simulink model "assgt4_friction"  (R2016a)
settings: Solver=VariableStepAuto  StartTime=0.0  StopTime=30  RelTol=1e-3
values from neighbouring files (symbols this model uses):
  g = 9.81    [assignment4.m]
  l1 = 1    [assignment4.m]
  l2 = 1    [assignment4.m]
  m1 = 1    [assignment4.m]
  m2 = 1    [assignment4.m]
  x_init = [-pi/2;0;0;0]    [assignment4.m]
undefined symbols (not defined in the file or in its folder): x
libraries: dspinverses x1
settings Model: Creator=Sondre  LastModifiedBy=Sondre

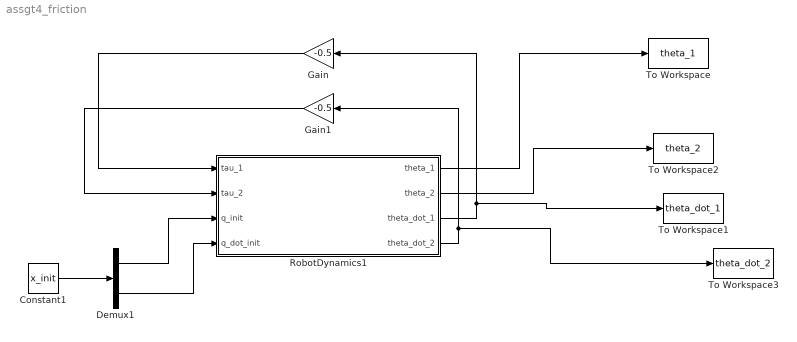
== system assgt4_friction ==
  Constant1 : Constant  Value=x_init
  Demux1 : Demux  Outputs=2
  Gain : Gain  Gain=-0.5
  Gain1 : Gain  Gain=-0.5
  RobotDynamics1 : Subsystem
  To Workspace : ToWorkspace  VariableName=theta_1  SaveFormat=Timeseries  SampleTime=-1
  To Workspace1 : ToWorkspace  VariableName=theta_dot_1  SaveFormat=Timeseries  SampleTime=-1
  To Workspace2 : ToWorkspace  VariableName=theta_2  SaveFormat=Timeseries  SampleTime=-1
  To Workspace3 : ToWorkspace  VariableName=theta_dot_2  SaveFormat=Timeseries  SampleTime=-1
  wires:
  RobotDynamics1/1(theta_1) -> To Workspace/1
  RobotDynamics1/2(theta_2) -> To Workspace2/1
  RobotDynamics1/3(theta_dot_1) -> Gain/1, To Workspace1/1
  RobotDynamics1/4(theta_dot_2) -> Gain1/1, To Workspace3/1
  Constant1/1 -> Demux1/1
  Demux1/1 -> RobotDynamics1/3(q_init)
  Demux1/2 -> RobotDynamics1/4(q_dot_init)
  Gain/1 -> RobotDynamics1/1(tau_1)
  Gain1/1 -> RobotDynamics1/2(tau_2)

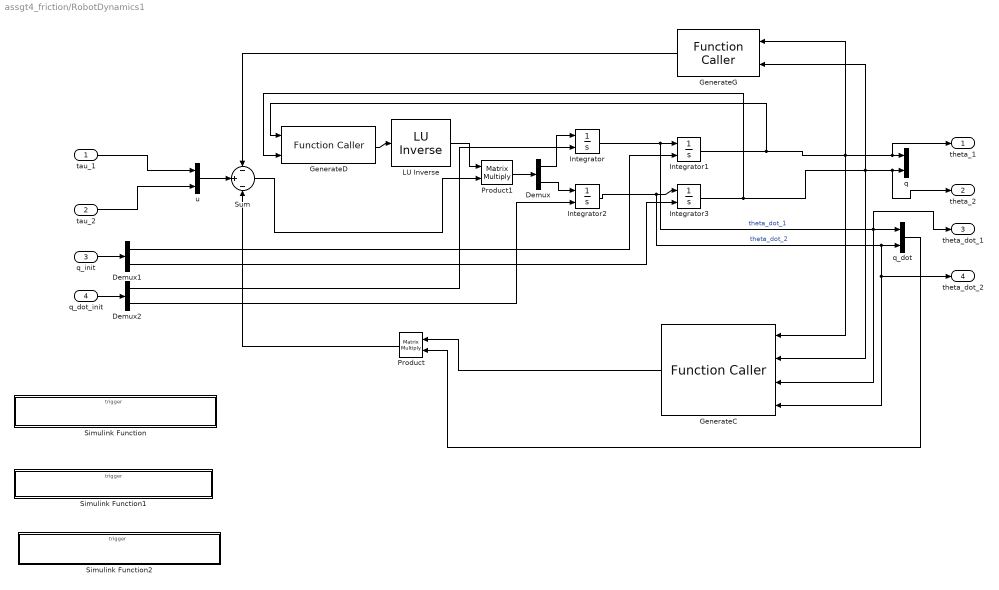
== system assgt4_friction/RobotDynamics1 ==
  tau_1 : Inport
  tau_2 : Inport  Port=2
  q_init : Inport  Port=3
  q_dot_init : Inport  Port=4
  " LU Inverse" : dspinverses/ LU Inverse
  Demux : Demux  Outputs=2
  Demux1 : Demux  Outputs=2
  Demux2 : Demux  Outputs=2
  GenerateC : FunctionCaller  FunctionPrototype=C = C(theta_1,theta_2,theta_dot_1,theta_dot_2)
  GenerateD : FunctionCaller  FunctionPrototype=D = D(theta_1,theta_2)
  GenerateG : FunctionCaller  FunctionPrototype=G = G(theta_1,theta_2)
  Integrator : Integrator  InitialConditionSource=external
  Integrator1 : Integrator  InitialConditionSource=external
  Integrator2 : Integrator  InitialConditionSource=external  InitialCondition=x(
  Integrator3 : Integrator  InitialConditionSource=external
  Product : Product  Multiplication=Matrix(*)
  Product1 : Product  Multiplication=Matrix(*)
  Simulink Function : Subsystem  TreatAsAtomicUnit=on
  Simulink Function1 : Subsystem  TreatAsAtomicUnit=on
  Simulink Function2 : Subsystem  TreatAsAtomicUnit=on
  Sum : Sum  Inputs=-|+|-
  q : Concatenate
  q_dot : Concatenate
  u : Concatenate
  theta_1 : Outport
  theta_2 : Outport  Port=2
  theta_dot_1 : Outport  Port=3
  theta_dot_2 : Outport  Port=4
  wires:
  tau_2/1 -> u/2
  tau_1/1 -> u/1
  u/1 -> Sum/2
  Product/1 -> Sum/3
  q_dot/1 -> Product/2
  GenerateG/1 -> Sum/1
  Sum/1 -> Product1/2
  GenerateC/1 -> Product/1
  GenerateD/1 -> " LU Inverse"/1
  " LU Inverse"/1 -> Product1/1
  Demux/1 -> Integrator/1
  Integrator/1 -> Integrator1/1, q_dot/1, GenerateC/3, theta_dot_1/1  "theta_dot_1"
  Demux/2 -> Integrator2/1
  Integrator2/1 -> GenerateC/4, theta_dot_2/1, q_dot/2, Integrator3/1  "theta_dot_2"
  Product1/1 -> Demux/1
  q_init/1 -> Demux1/1
  q_dot_init/1 -> Demux2/1
  Demux2/1 -> Integrator/2
  Demux2/2 -> Integrator2/2
  Demux1/1 -> Integrator1/2
  Demux1/2 -> Integrator3/2
  Integrator1/1 -> GenerateD/1, theta_1/1, q/1, GenerateG/1, GenerateC/1
  Integrator3/1 -> GenerateD/2, GenerateC/2, GenerateG/2, theta_2/1, q/2

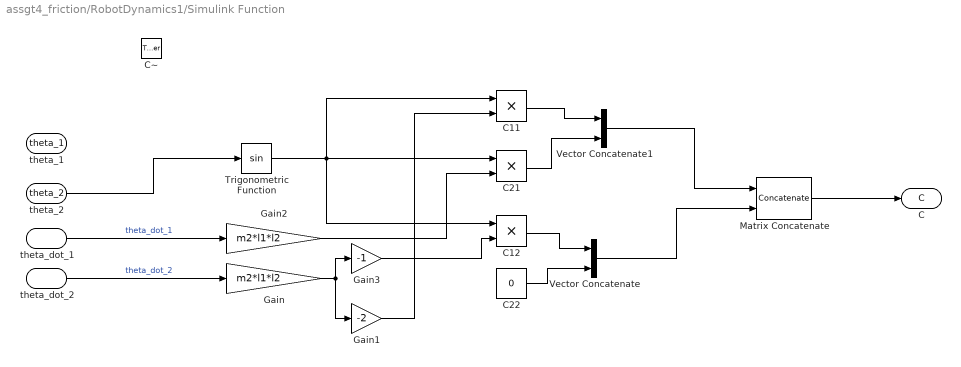
== system assgt4_friction/RobotDynamics1/Simulink Function ==
  C~ : TriggerPort  TriggerType=function-call  IsSimulinkFunction=on  FunctionName=C  VariantControl=Variant
  C11 : Product
  C12 : Product
  C21 : Product
  C22 : Constant  Value=0
  Gain : Gain  Gain=m2*l1*l2
  Gain1 : Gain  Gain=-2
  Gain2 : Gain  Gain=m2*l1*l2
  Gain3 : Gain  Gain=-1
  Matrix Concatenate : Concatenate  Mode=Multidimensional array  ConcatenateDimension=2
  Trigonometric Function : Trigonometry
  Vector Concatenate : Concatenate
  Vector Concatenate1 : Concatenate
  theta_1 : ArgIn  DisableCoverage=on  ArgumentName=theta_1
  theta_2 : ArgIn  DisableCoverage=on  Port=2  ArgumentName=theta_2
  theta_dot_1 : ArgIn  DisableCoverage=on  Port=3  ArgumentName=theta_dot_1
  theta_dot_2 : ArgIn  DisableCoverage=on  Port=4  ArgumentName=theta_dot_2
  C : ArgOut  DisableCoverage=on  PortDimensions=[2 2]  ArgumentName=C
  wires:
  theta_dot_1/1 -> Gain2/1  "theta_dot_1"
  theta_dot_2/1 -> Gain/1  "theta_dot_2"
  Trigonometric Function/1 -> C12/1, C11/1, C21/1
  C11/1 -> Vector Concatenate1/1
  Gain/1 -> Gain3/1, Gain1/1
  Gain1/1 -> C11/2
  C21/1 -> Vector Concatenate1/2
  Gain2/1 -> C21/2
  Gain3/1 -> C12/2
  C12/1 -> Vector Concatenate/1
  C22/1 -> Vector Concatenate/2
  theta_2/1 -> Trigonometric Function/1
  Matrix Concatenate/1 -> C/1
  Vector Concatenate1/1 -> Matrix Concatenate/1
  Vector Concatenate/1 -> Matrix Concatenate/2

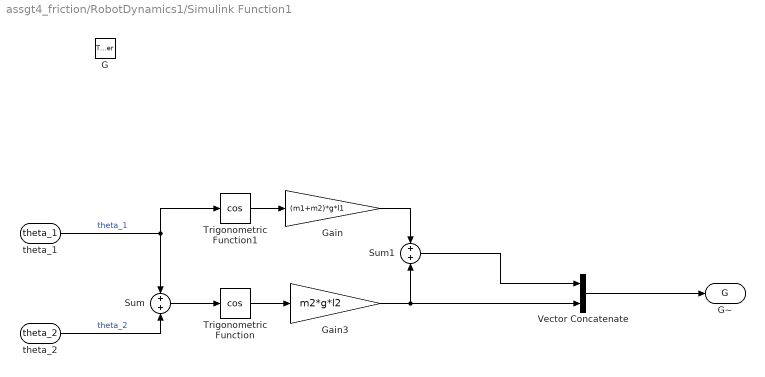
== system assgt4_friction/RobotDynamics1/Simulink Function1 ==
  G : TriggerPort  TriggerType=function-call  IsSimulinkFunction=on  FunctionName=G  VariantControl=Variant
  Gain : Gain  Gain=(m1+m2)*g*l1
  Gain3 : Gain  Gain=m2*g*l2
  Sum : Sum  Inputs=+|+
  Sum1 : Sum  Inputs=+|+
  Trigonometric Function : Trigonometry  Operator=cos
  Trigonometric Function1 : Trigonometry  Operator=cos
  Vector Concatenate : Concatenate
  theta_1 : ArgIn  DisableCoverage=on  ArgumentName=theta_1
  theta_2 : ArgIn  DisableCoverage=on  Port=2  ArgumentName=theta_2
  G~ : ArgOut  DisableCoverage=on  PortDimensions=[2 1]  ArgumentName=G
  wires:
  theta_1/1 -> Trigonometric Function1/1, Sum/1  "theta_1"
  theta_2/1 -> Sum/2  "theta_2"
  Sum/1 -> Trigonometric Function/1
  Vector Concatenate/1 -> G~/1
  Trigonometric Function1/1 -> Gain/1
  Trigonometric Function/1 -> Gain3/1
  Gain/1 -> Sum1/1
  Gain3/1 -> Sum1/2, Vector Concatenate/2
  Sum1/1 -> Vector Concatenate/1

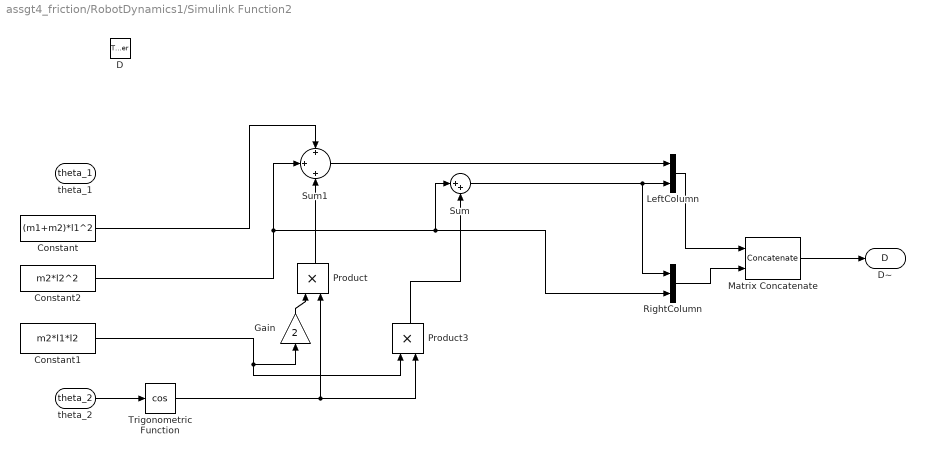
== system assgt4_friction/RobotDynamics1/Simulink Function2 ==
  D : TriggerPort  TriggerType=function-call  IsSimulinkFunction=on  FunctionName=D  VariantControl=Variant
  Constant : Constant  Value=(m1+m2)*l1^2
  Constant1 : Constant  Value=m2*l1*l2
  Constant2 : Constant  Value=m2*l2^2
  Gain : Gain  Gain=2
  LeftColumn : Concatenate
  Matrix Concatenate : Concatenate  Mode=Multidimensional array  ConcatenateDimension=2
  Product : Product
  Product3 : Product
  RightColumn : Concatenate
  Sum : Sum  Inputs=|++
  Sum1 : Sum  Inputs=+|+|+
  Trigonometric Function : Trigonometry  Operator=cos
  theta_1 : ArgIn  DisableCoverage=on  ArgumentName=theta_1
  theta_2 : ArgIn  DisableCoverage=on  Port=2  ArgumentName=theta_2
  D~ : ArgOut  DisableCoverage=on  PortDimensions=[2 2]  ArgumentName=D
  wires:
  theta_2/1 -> Trigonometric Function/1
  Matrix Concatenate/1 -> D~/1
  Constant1/1 -> Gain/1, Product3/1
  Gain/1 -> Product/1
  Product/1 -> Sum1/3
  Constant/1 -> Sum1/1
  Constant2/1 -> Sum1/2, RightColumn/2, Sum/1
  Sum1/1 -> LeftColumn/1
  Product3/1 -> Sum/2
  Trigonometric Function/1 -> Product/2, Product3/2
  Sum/1 -> RightColumn/1, LeftColumn/2
  LeftColumn/1 -> Matrix Concatenate/1
  RightColumn/1 -> Matrix Concatenate/2
